simulink library "utils"  (R2014b)
settings: Solver=ode45  StartTime=0.0  StopTime=10.0  RelTol=1e-3
settings Model: Creator=Meyer-Brügel  LastModifiedBy=Meyer-Brügel

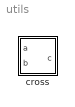
== system utils ==
  "cross " : Subsystem  TreatAsAtomicUnit=on

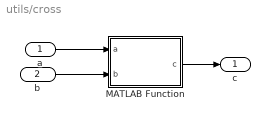
== system utils/cross  ==
  a : Inport  PortDimensions=[3,1]
  b : Inport  Port=2  PortDimensions=[3,1]
  MATLAB Function : MATLAB Function  TreatAsAtomicUnit=on
  c : Outport  PortDimensions=[3,1]
  wires:
  b/1 -> MATLAB Function/2(b)
  a/1 -> MATLAB Function/1(a)
  MATLAB Function/1(c) -> c/1

== matlab function utils/cross /MATLAB Function ==
  data: a input size=[3,1]; c output size=[3,1]; b input size=[3,1]
function c = fcn(a,b)
%#codegen

c=cross(a,b);
